simulink model "exp05"  (R2020b)
settings: Solver=VariableStepAuto  StartTime=0.0  StopTime=10.0  RelTol=1e-3
settings Model: Creator=1  LastModifiedBy=1

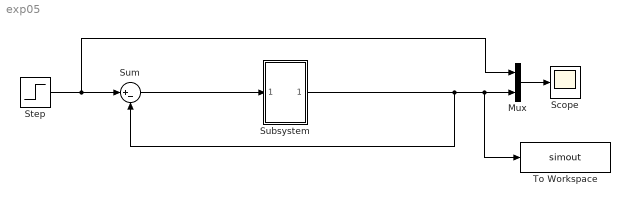
== system exp05 ==
  Mux : Mux  Inputs=2
  Scope : Scope
  Step : Step  SampleTime=0
  Subsystem : Subsystem
  Sum : Sum  Inputs=|+-
  To Workspace : ToWorkspace  VariableName=simout  SaveFormat=Timeseries  SampleTime=-1
  wires:
  Subsystem/1(Out1) -> To Workspace/1, Mux/2, Sum/2
  Sum/1 -> Subsystem/1(In1)
  Step/1 -> Mux/1, Sum/1
  Mux/1 -> Scope/1

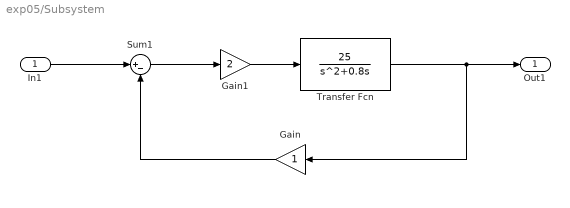
== system exp05/Subsystem ==
  In1 : Inport
  Gain : Gain
  Gain1 : Gain  Gain=2
  Sum1 : Sum  Inputs=|+-
  Transfer Fcn : TransferFcn  Numerator=[0 0 25]  Denominator=[1 0.8 0]
  Out1 : Outport
  wires:
  In1/1 -> Sum1/1
  Transfer Fcn/1 -> Gain/1, Out1/1
  Gain1/1 -> Transfer Fcn/1
  Gain/1 -> Sum1/2
  Sum1/1 -> Gain1/1
